simulink model "CM012A_FordT3McuCfg"  (R2013b)
settings: Solver=FixedStepDiscrete  SolverMode=SingleTasking  StartTime=0.0  StopTime=2  FixedStep=0.00005  RelTol=1e-3
values from neighbouring files (symbols this model uses):
  BATTVLTGSCAGFAC_ULS_F32 = DataDict.Constant    [CM012A_FordT3McuCfg_DataDict.m]
  BATTVLTGSWD1SCAGFAC_ULS_F32 = DataDict.Constant    [CM012A_FordT3McuCfg_DataDict.m]
  CHRGPMPDIAGSCAGFAC_ULS_F32 = DataDict.Constant    [CM012A_FordT3McuCfg_DataDict.m]
  MOTAG2MEAS_ECU1OFFS_MOTREV_F32 = DataDict.Constant    [CM012A_FordT3McuCfg_DataDict.m]
  MOTAG2MEAS_ECU2OFFS_MOTREV_F32 = DataDict.Constant    [CM012A_FordT3McuCfg_DataDict.m]
  PWRDISCNCTSWTDIAGSCAGFAC_ULS_F32 = DataDict.Constant    [CM012A_FordT3McuCfg_DataDict.m]
undefined symbols (not defined in the file or in its folder): HwAgSnsrTyp1, sigbuilder_block
libraries: CM012A_FordT3McuCfg_ModelLibrary x114, simulink x37, NxtrLim x34
(part 2 of 4)

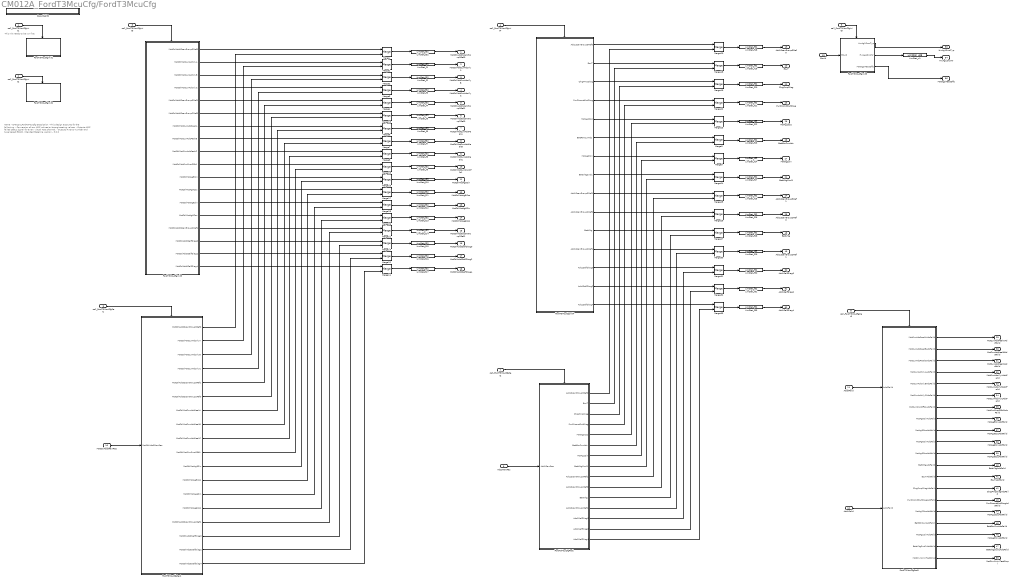
== system CM012A_FordT3McuCfg/FordT3McuCfg ==
  note: Name - 		CM012A_FordT3McuCfg
      | Description -  This design accounts for the following,
      | 			- Conversion of raw ADC values to its engineering values.
      | 			- Outputs ADC failed status signal for every virtual ADC channel.
      | 			- Outputs HwSnsr number and type based ECUID.
      | Intended Baseline version - 3.0.0
  note: This Init needs to be run first
  call_FordT3McuCfgInit1 : Inport
  call_FordT3McuCfgInit2 : Inport  Port=2
  call_FordT3McuCfgInit3 : Inport  Port=3
  call_FordT3McuCfgInit4 : Inport  Port=4
  call_FordT3McuCfgInit5 : Inport  Port=5
  call_FordT3McuCfgPer1 : Inport  Port=6
  call_FordT3McuCfgPer2 : Inport  Port=7
  call_FordT3McuCfgPer3 : Inport  Port=8
  Adc1RawRes : Inport  RequirementInfo="{'linktype_rmi_doors' '00016ba8 (/ESG Group/FDD Module Requirements/EA4 Specific/CM012A_FordT3McuCfg)' '#CM012A_80' 'true' 'REQ:  CM012A_80' '' } %GIDa_41160691_1e7a_406c_957b_4d6a456ee094"  Port=9
  MotCtrlAdc0RawRes : Inport  RequirementInfo="{'linktype_rmi_doors' '00016ba8 (/ESG Group/FDD Module Requirements/EA4 Specific/CM012A_FordT3McuCfg)' '#CM012A_30' 'true' 'REQ:  CM012A_30' '' } %GIDa_99229d35_45d9_4e08_a805_76e263dac1ca"  Port=10
  Adc0Faild : Inport  RequirementInfo="{'linktype_rmi_doors' '00016ba8 (/ESG Group/FDD Module Requirements/EA4 Specific/CM012A_FordT3McuCfg)' '#CM012A_108' 'true' 'REQ:  CM012A_108' '' } %GIDa_0bce0144_3b89_427c_817c_6b44de9e7a17"  Port=11
  Adc1Faild : Inport  RequirementInfo="{'linktype_rmi_doors' '00016ba8 (/ESG Group/FDD Module Requirements/EA4 Specific/CM012A_FordT3McuCfg)' '#CM012A_109' 'true' 'REQ:  CM012A_109' '' } %GIDa_dca9ee74_b82a_443a_9b96_53a5f3cd54c7"  Port=12
  EcuId : Inport  RequirementInfo="{'linktype_rmi_doors' '00016ba8 (/ESG Group/FDD Module Requirements/EA4 Specific/CM012A_FordT3McuCfg)' '#CM012A_110' 'true' 'REQ:  CM012A_110' '' } %GIDa_2ea2a6bb_1285_46d2_bb52_886e41c9a838"  Port=13
  CopyRight2 : Subsystem  Description=|  mask(Copyright Information){none=on}
      | Copyright info block.                                               
      |                                                                     
      | Place copyright information at the top of every subsystem in design.
      mask prompts: none "No parameters"
      mask help: Place copyright information at the top of every subsystem in design.
      mask Display:
      | NxtrConf = 'Nexteer Confidential';
      | 
      | sys = bdroot; %handle for the current model ("system")
      | first = get_param(sys,'Created');
      | first = first(end-3:end);  %year is last four digits
      | 
      | last = get_param(sys,'LastModifiedDate');
      | if isempty(last)
      |     last = datestr(now,'yyyy');
      | else
      |     last = last(end-3:end);
      | end
      | 
      | if strcmp(first,last)
      |     fprintf('%s -- Copyright %s Nexteer',NxtrConf,first)
      | else
      |     fprintf('%s -- %s%s- %s Nexteer',NxtrConf,char(169),first,last)
      | end
  FordT3McuCfgInit1 : Subsystem
  FordT3McuCfgInit2 : Subsystem
  FordT3McuCfgInit3 : Subsystem
  FordT3McuCfgInit4 : Subsystem
  FordT3McuCfgInit5 : Subsystem  RequirementInfo="{'linktype_rmi_doors' '00016ba8 (/ESG Group/FDD Module Requirements/EA4 Specific/CM012A_FordT3McuCfg)' '#CM012A_188' 'true' 'REQ:  CM012A_188' '' } %GIDa_a4501015_2e8d_4379_8b64_871cd7f02fc6"
  FordT3McuCfgPer1 : Subsystem  RequirementInfo="{'linktype_rmi_doors' '00016ba8 (/ESG Group/FDD Module Requirements/EA4 Specific/CM012A_FordT3McuCfg)' '#CM012A_113' 'true' 'REQ:  CM012A_113' '' } %GIDa_f4084d5f_812f_4f7b_9c4a_edd3fedcd563"
      settings: AttributesFormatString=Priority: %<Priority>
  FordT3McuCfgPer2 : Subsystem  RequirementInfo="{'linktype_rmi_doors' '00016ba8 (/ESG Group/FDD Module Requirements/EA4 Specific/CM012A_FordT3McuCfg)' '#CM012A_114' 'true' 'REQ:  CM012A_114' '' } %GIDa_f8eec309_27b4_4df0_b18c_c2951f94362c"
      settings: AttributesFormatString=Priority: %<Priority>
  FordT3McuCfgPer3 : Subsystem  RequirementInfo="{'linktype_rmi_doors' '00016ba8 (/ESG Group/FDD Module Requirements/EA4 Specific/CM012A_FordT3McuCfg)' '#CM012A_134' 'true' 'REQ:  CM012A_134' '' } %GIDa_f61b09d0_e9f4_4379_bee3_c878705b543d"
      settings: AttributesFormatString=Priority: %<Priority>
  LimStat_f{1..19,22..26,29..33} (29 alike) : NxtrLim/LimStat_f32  LoLim=0  HiLim=ADCOUTPMAX_VOLT_F32
      settings: AttributesFormatString=|
      | Low Limit: %<LoLim>
      | High Limit:%<HiLim>
  LimStat_f{20..21,27..28} (4 alike) : NxtrLim/LimStat_f32  LoLim=0  HiLim=BATTADCOUTPMAX_VOLT_F32
      settings: AttributesFormatString=|
      | Low Limit: %<LoLim>
      | High Limit:%<HiLim>
  LimStat_u1 : NxtrLim/LimStat_u08  LoLim=0  HiLim=HWAG1SNSRNRMAX_CNT_F32
      settings: AttributesFormatString=|
      | Low Limit: %<LoLim>
      | High Limit:%<HiLim>
  Merge{,1..9,11..33} (33 alike) : Merge
  MotCtrlAdc0ScanGroup3Ref0 : Outport
  MotCtrlMotCurrAdcVlyA : Outport  RequirementInfo="{'linktype_rmi_doors' '00016ba8 (/ESG Group/FDD Module Requirements/EA4 Specific/CM012A_FordT3McuCfg)' '#CM012A_31' 'true' 'REQ:  CM012A_31' '' } %GIDa_0bdba440_75b6_48b6_84a8_aedbc0ed0aee"  Port=2
  MotCtrlMotCurrAdcVlyB : Outport  RequirementInfo="{'linktype_rmi_doors' '00016ba8 (/ESG Group/FDD Module Requirements/EA4 Specific/CM012A_FordT3McuCfg)' '#CM012A_97' 'true' 'REQ:  CM012A_97' '' } %GIDa_ce9d7107_8d39_410b_aef3_5c211a563983"  Port=3
  MotCtrlMotCurrAdcVlyC : Outport  RequirementInfo="{'linktype_rmi_doors' '00016ba8 (/ESG Group/FDD Module Requirements/EA4 Specific/CM012A_FordT3McuCfg)' '#CM012A_96' 'true' 'REQ:  CM012A_96' '' } %GIDa_d8883527_c83e_4baa_9ea4_71e3d2339800"  Port=4
  MotCtrlAdc0ScanGroup3Ref1 : Outport  Port=5
  MotCtrlAdc0ScanGroup2Ref0 : Outport  Port=6
  MotCtrlMotCurrAdcPeakA : Outport  RequirementInfo="{'linktype_rmi_doors' '00016ba8 (/ESG Group/FDD Module Requirements/EA4 Specific/CM012A_FordT3McuCfg)' '#CM012A_135' 'true' 'REQ:  CM012A_135' '' } %GIDa_3269826c_f262_49f9_8a60_4071384b86b7"  Port=7
  MotCtrlMotCurrAdcPeakB : Outport  RequirementInfo="{'linktype_rmi_doors' '00016ba8 (/ESG Group/FDD Module Requirements/EA4 Specific/CM012A_FordT3McuCfg)' '#CM012A_136' 'true' 'REQ:  CM012A_136' '' } %GIDa_7e88d78e_c6ec_4e32_98f2_6110e77972ae"  Port=8
  MotCtrlMotCurrAdcPeakC : Outport  RequirementInfo="{'linktype_rmi_doors' '00016ba8 (/ESG Group/FDD Module Requirements/EA4 Specific/CM012A_FordT3McuCfg)' '#CM012A_137' 'true' 'REQ:  CM012A_137' '' } %GIDa_58277148_ccdb_4560_8c9d_d26260a4df88"  Port=9
  MotCtrlMotCurrSnsrOffs1 : Outport  RequirementInfo="{'linktype_rmi_doors' '00016ba8 (/ESG Group/FDD Module Requirements/EA4 Specific/CM012A_FordT3McuCfg)' '#CM012A_138' 'true' 'REQ:  CM012A_138' '' } %GIDa_8dfc8efb_0597_44a1_ac28_cdaba55153cb"  Port=10
  MotCtrlMotAg5Sin : Outport  RequirementInfo="{'linktype_rmi_doors' '00016ba8 (/ESG Group/FDD Module Requirements/EA4 Specific/CM012A_FordT3McuCfg)' '#CM012A_139' 'true' 'REQ:  CM012A_139' '' } %GIDa_8814a36d_2960_4cab_9305_7cef514a95a4"  Port=11
  MotCtrlMotAg5Cos : Outport  RequirementInfo="{'linktype_rmi_doors' '00016ba8 (/ESG Group/FDD Module Requirements/EA4 Specific/CM012A_FordT3McuCfg)' '#CM012A_140' 'true' 'REQ:  CM012A_140' '' } %GIDa_cf319651_e51f_428f_a8b0_82c784d893cb"  Port=12
  MotCtrlMotAg6Sin : Outport  RequirementInfo="{'linktype_rmi_doors' '00016ba8 (/ESG Group/FDD Module Requirements/EA4 Specific/CM012A_FordT3McuCfg)' '#CM012A_141' 'true' 'REQ:  CM012A_141' '' } %GIDa_f3249900_9d1e_416f_98e2_ff7658e30e7b"  Port=13
  MotCtrlMotAg6Cos : Outport  RequirementInfo="{'linktype_rmi_doors' '00016ba8 (/ESG Group/FDD Module Requirements/EA4 Specific/CM012A_FordT3McuCfg)' '#CM012A_142' 'true' 'REQ:  CM012A_142' '' } %GIDa_bed7064b_f1cf_47a3_89f1_2e6806942a9b"  Port=14
  MotCtrlAdc0ScanGroup2Ref1 : Outport  Port=15
  MotCtrlAdc0SelfDiag0 : Outport  Port=16
  MotCtrlAdc0SelfDiag2 : Outport  Port=17
  MotCtrlAdc0SelfDiag4 : Outport  Port=18
  Adc1ScanGroup3Ref0 : Outport  Port=19
  EcuT : Outport  RequirementInfo="{'linktype_rmi_doors' '00016ba8 (/ESG Group/FDD Module Requirements/EA4 Specific/CM012A_FordT3McuCfg)' '#CM012A_143' 'true' 'REQ:  CM012A_143' '' } %GIDa_4e0089fd_73ae_4216_9e55_f5e900769cc9"  Port=20
  BattVltgSwd1 : Outport  RequirementInfo="{'linktype_rmi_doors' '00016ba8 (/ESG Group/FDD Module Requirements/EA4 Specific/CM012A_FordT3McuCfg)' '#CM012A_148' 'true' 'REQ:  CM012A_148' '' } %GIDa_a4fbd9dd_cc02_44b6_8c60_edd2cbad70c3"  Port=21
  ChrgPmpDiag : Outport  RequirementInfo="{'linktype_rmi_doors' '00016ba8 (/ESG Group/FDD Module Requirements/EA4 Specific/CM012A_FordT3McuCfg)' '#CM012A_144' 'true' 'REQ:  CM012A_144' '' } %GIDa_9af4aaf1_e6d4_4150_aa90_b727a20d0e65"  Port=22
  PwrDiscnctSwtDiag : Outport  RequirementInfo="{'linktype_rmi_doors' '00016ba8 (/ESG Group/FDD Module Requirements/EA4 Specific/CM012A_FordT3McuCfg)' '#CM012A_186' 'true' 'REQ:  CM012A_186' '' } %GIDa_25930d50_606d_4173_986f_d131b07fb4a3"  Port=23
  Adc1ScanGroup3Ref1 : Outport  Port=24
  Adc1ScanGroup2Ref0 : Outport  Port=25
  MotAg2Cos : Outport  RequirementInfo="{'linktype_rmi_doors' '00016ba8 (/ESG Group/FDD Module Requirements/EA4 Specific/CM012A_FordT3McuCfg)' '#CM012A_145' 'true' 'REQ:  CM012A_145' '' } %GIDa_fb1722b1_4d2c_4680_9aaf_1a870d66429d"  Port=26
  MotAg2Sin : Outport  RequirementInfo="{'linktype_rmi_doors' '00016ba8 (/ESG Group/FDD Module Requirements/EA4 Specific/CM012A_FordT3McuCfg)' '#CM012A_147' 'true' 'REQ:  CM012A_147' '' } %GIDa_119a92d6_b549_4670_801c_893abfbf86fb"  Port=27
  BattRtnCurrAdc : Outport  RequirementInfo="{'linktype_rmi_doors' '00016ba8 (/ESG Group/FDD Module Requirements/EA4 Specific/CM012A_FordT3McuCfg)' '#CM012A_146' 'true' 'REQ:  CM012A_146' '' } %GIDa_bf47c31e_57b3_45f9_b1b7_bf963f3d70ff"  Port=28
  MotCurrAdcPeakAAdcFaild : Outport  RequirementInfo="{'linktype_rmi_doors' '00016ba8 (/ESG Group/FDD Module Requirements/EA4 Specific/CM012A_FordT3McuCfg)' '#CM012A_149' 'true' 'REQ:  CM012A_149' '' } %GIDa_3a53e3dd_f880_4695_94e7_22bc9fe6702f"  Port=29
  MotCurrAdcPeakBAdcFaild : Outport  RequirementInfo="{'linktype_rmi_doors' '00016ba8 (/ESG Group/FDD Module Requirements/EA4 Specific/CM012A_FordT3McuCfg)' '#CM012A_150' 'true' 'REQ:  CM012A_150' '' } %GIDa_feafdf78_53ff_40fe_9421_17b92296df86"  Port=30
  MotCurrAdcPeakCAdcFaild : Outport  RequirementInfo="{'linktype_rmi_doors' '00016ba8 (/ESG Group/FDD Module Requirements/EA4 Specific/CM012A_FordT3McuCfg)' '#CM012A_151' 'true' 'REQ:  CM012A_151' '' } %GIDa_56e34d84_3367_4a32_8cb7_70a413310ee9"  Port=31
  MotCurrAdcVlyAAdcFaild : Outport  RequirementInfo="{'linktype_rmi_doors' '00016ba8 (/ESG Group/FDD Module Requirements/EA4 Specific/CM012A_FordT3McuCfg)' '#CM012A_152' 'true' 'REQ:  CM012A_152' '' } %GIDa_235f97ec_d780_48fb_a6ee_f7442017c90d"  Port=32
  MotCurrAdcVlyBAdcFaild : Outport  RequirementInfo="{'linktype_rmi_doors' '00016ba8 (/ESG Group/FDD Module Requirements/EA4 Specific/CM012A_FordT3McuCfg)' '#CM012A_153' 'true' 'REQ:  CM012A_153' '' } %GIDa_353b0153_747a_4ed6_88df_12a4ad6b71ec"  Port=33
  MotCurrAdcVlyCAdcFaild : Outport  RequirementInfo="{'linktype_rmi_doors' '00016ba8 (/ESG Group/FDD Module Requirements/EA4 Specific/CM012A_FordT3McuCfg)' '#CM012A_154' 'true' 'REQ:  CM012A_154' '' } %GIDa_a57b872d_9b77_463d_8457_590115cc1f58"  Port=34
  MotCurrSnsrOffs1AdcFaild : Outport  RequirementInfo="{'linktype_rmi_doors' '00016ba8 (/ESG Group/FDD Module Requirements/EA4 Specific/CM012A_FordT3McuCfg)' '#CM012A_155' 'true' 'REQ:  CM012A_155' '' } %GIDa_dab1b948_9138_4007_9c31_06f0147cb8f7"  Port=35
  MotAg5SinAdcFaild : Outport  RequirementInfo="{'linktype_rmi_doors' '00016ba8 (/ESG Group/FDD Module Requirements/EA4 Specific/CM012A_FordT3McuCfg)' '#CM012A_156' 'true' 'REQ:  CM012A_156' '' } %GIDa_0b267258_9b4b_4074_b8ac_2e562917866b"  Port=36
  MotAg5CosAdcFaild : Outport  RequirementInfo="{'linktype_rmi_doors' '00016ba8 (/ESG Group/FDD Module Requirements/EA4 Specific/CM012A_FordT3McuCfg)' '#CM012A_157' 'true' 'REQ:  CM012A_157' '' } %GIDa_2a7f7a18_8db2_45e1_a969_e1b831e06969"  Port=37
  MotAg6SinAdcFaild : Outport  RequirementInfo="{'linktype_rmi_doors' '00016ba8 (/ESG Group/FDD Module Requirements/EA4 Specific/CM012A_FordT3McuCfg)' '#CM012A_158' 'true' 'REQ:  CM012A_158' '' } %GIDa_5066297d_e1ca_466f_b5fd_4f065ba4d243"  Port=38
  MotAg6CosAdcFaild : Outport  RequirementInfo="{'linktype_rmi_doors' '00016ba8 (/ESG Group/FDD Module Requirements/EA4 Specific/CM012A_FordT3McuCfg)' '#CM012A_159' 'true' 'REQ:  CM012A_159' '' } %GIDa_42b69db8_ef47_41c4_a15d_6b9505077de8"  Port=39
  BattVltgAdcFaild : Outport  RequirementInfo="{'linktype_rmi_doors' '00016ba8 (/ESG Group/FDD Module Requirements/EA4 Specific/CM012A_FordT3McuCfg)' '#CM012A_160' 'true' 'REQ:  CM012A_160' '' } %GIDa_f2237051_f0a5_4ae7_a3b8_c07d1c352a88"  Port=40
  EcuTAdcFaild : Outport  RequirementInfo="{'linktype_rmi_doors' '00016ba8 (/ESG Group/FDD Module Requirements/EA4 Specific/CM012A_FordT3McuCfg)' '#CM012A_161' 'true' 'REQ:  CM012A_161' '' } %GIDa_f8c196a4_34a8_4792_9bba_d1d568e93057"  Port=41
  ChrgPmpDiagAdcFaild : Outport  RequirementInfo="{'linktype_rmi_doors' '00016ba8 (/ESG Group/FDD Module Requirements/EA4 Specific/CM012A_FordT3McuCfg)' '#CM012A_162' 'true' 'REQ:  CM012A_162' '' } %GIDa_77beee14_d374_44df_95fc_54a895c9cfa9"  Port=42
  PwrDiscnctSwtDiagAdcFaild : Outport  RequirementInfo="{'linktype_rmi_doors' '00016ba8 (/ESG Group/FDD Module Requirements/EA4 Specific/CM012A_FordT3McuCfg)' '#CM012A_163' 'true' 'REQ:  CM012A_163' '' } %GIDa_31860440_5fb5_4509_8c25_9f6b0fdcba7a"  Port=43
  MotAg2CosAdcFaild : Outport  RequirementInfo="{'linktype_rmi_doors' '00016ba8 (/ESG Group/FDD Module Requirements/EA4 Specific/CM012A_FordT3McuCfg)' '#CM012A_164' 'true' 'REQ:  CM012A_164' '' } %GIDa_a152779b_3d52_4dd5_9e9f_688e8ab12150"  Port=44
  BattRtnCurrAdcFaild : Outport  RequirementInfo="{'linktype_rmi_doors' '00016ba8 (/ESG Group/FDD Module Requirements/EA4 Specific/CM012A_FordT3McuCfg)' '#CM012A_165' 'true' 'REQ:  CM012A_165' '' } %GIDa_209c41ad_d5d9_4f94_9c3e_4b63790d466d"  Port=45
  MotAg2SinAdcFaild : Outport  RequirementInfo="{'linktype_rmi_doors' '00016ba8 (/ESG Group/FDD Module Requirements/EA4 Specific/CM012A_FordT3McuCfg)' '#CM012A_166' 'true' 'REQ:  CM012A_166' '' } %GIDa_2107ec05_8c9a_4950_b739_abe494ef6948"  Port=46
  BattVltgSwd1AdcFaild : Outport  RequirementInfo="{'linktype_rmi_doors' '00016ba8 (/ESG Group/FDD Module Requirements/EA4 Specific/CM012A_FordT3McuCfg)' '#CM012A_167' 'true' 'REQ:  CM012A_167' '' } %GIDa_c3b1591d_1c63_48f3_97b0_16e822f187b4"  Port=47
  BattVltg : Outport  RequirementInfo="{'linktype_rmi_doors' '00016ba8 (/ESG Group/FDD Module Requirements/EA4 Specific/CM012A_FordT3McuCfg)' '#CM012A_187' 'true' 'REQ:  CM012A_187' '' } %GIDa_e1d6f2ac_b011_4b4e_acb7_aa6bb65164ac"  Port=48
  Adc1ScanGroup2Ref1 : Outport  Port=49
  Adc1SelfDiag0 : Outport  Port=50
  Adc1SelfDiag2 : Outport  Port=51
  Adc1SelfDiag4 : Outport  Port=52
  HwAg1SnsrTyp : Outport  RequirementInfo="{'linktype_rmi_doors' '00016ba8 (/ESG Group/FDD Module Requirements/EA4 Specific/CM012A_FordT3McuCfg)' '#CM012A_168' 'true' 'REQ:  CM012A_168' '' } %GIDa_345868f1_11a8_4efe_8557_e97fce4612b7"  Port=53
  HwAg1SnsrNr : Outport  RequirementInfo="{'linktype_rmi_doors' '00016ba8 (/ESG Group/FDD Module Requirements/EA4 Specific/CM012A_FordT3McuCfg)' '#CM012A_169' 'true' 'REQ:  CM012A_169' '' } %GIDa_0d5e4ab3_9e68_4afd_8e94_0b3421e961a0"  Port=54
  MotDrvr1IninTestCmpl : Outport  Port=55
  MotAg2MeasOffs : Outport  RequirementInfo="{'linktype_rmi_doors' '00016ba8 (/ESG Group/FDD Module Requirements/EA4 Specific/CM012A_FordT3McuCfg)' '#CM012A_192' 'true' 'REQ:  CM012A_192' '' } %GIDa_2a555be6_74a0_4831_8830_82a88131d4c1"  Port=56
  wires:
  FordT3McuCfgInit3/1(MotCtrlAdc0ScanGroup3Ref0) -> Merge/1
  FordT3McuCfgInit3/2(MotCtrlMotCurrAdcVlyA) -> Merge1/1
  FordT3McuCfgInit3/3(MotCtrlMotCurrAdcVlyB) -> Merge2/1
  FordT3McuCfgInit3/4(MotCtrlMotCurrAdcVlyC) -> Merge3/1
  FordT3McuCfgInit3/5(MotCtrlAdc0ScanGroup3Ref1) -> Merge4/1
  FordT3McuCfgInit3/6(MotCtrlAdc0ScanGroup2Ref0) -> Merge13/1
  FordT3McuCfgInit3/7(MotCtrlMotCurrAdcPeakA) -> Merge6/1
  FordT3McuCfgInit3/8(MotCtrlMotCurrAdcPeakB) -> Merge7/1
  FordT3McuCfgInit3/9(MotCtrlMotCurrAdcPeakC) -> Merge8/1
  FordT3McuCfgInit3/10(MotCtrlMotCurrSnsrOffs1) -> Merge15/1
  FordT3McuCfgInit3/11(MotCtrlMotAg5Sin) -> Merge16/1
  FordT3McuCfgInit3/12(MotCtrlMotAg5Cos) -> Merge17/1
  FordT3McuCfgInit3/13(MotCtrlMotAg6Sin) -> Merge28/1
  FordT3McuCfgInit3/14(MotCtrlMotAg6Cos) -> Merge26/1
  FordT3McuCfgInit3/15(MotCtrlAdc0ScanGroup2Ref1) -> Merge21/1
  FordT3McuCfgInit3/16(MotCtrlAdc0SelfDiag0) -> Merge14/1
  FordT3McuCfgInit3/17(MotCtrlAdc0SelfDiag2) -> Merge12/1
  FordT3McuCfgInit3/18(MotCtrlAdc0SelfDiag4) -> Merge11/1
  FordT3McuCfgPer1/18(MotCtrlAdc0SelfDiag4) -> Merge11/2
  FordT3McuCfgPer1/17(MotCtrlAdc0SelfDiag2) -> Merge12/2
  FordT3McuCfgPer1/16(MotCtrlAdc0SelfDiag0) -> Merge14/2
  FordT3McuCfgPer1/15(MotCtrlAdc0ScanGroup2Ref1) -> Merge21/2
  FordT3McuCfgPer1/14(MotCtrlMotAg6Cos) -> Merge26/2
  FordT3McuCfgPer1/13(MotCtrlMotAg6Sin) -> Merge28/2
  FordT3McuCfgPer1/12(MotCtrlMotAg5Cos) -> Merge17/2
  FordT3McuCfgPer1/11(MotCtrlMotAg5Sin) -> Merge16/2
  FordT3McuCfgPer1/10(MotCtrlMotCurrSnsrOffs1) -> Merge15/2
  FordT3McuCfgPer1/9(MotCtrlMotCurrAdcPeakC) -> Merge8/2
  FordT3McuCfgPer1/8(MotCtrlMotCurrAdcPeakB) -> Merge7/2
  FordT3McuCfgPer1/7(MotCtrlMotCurrAdcPeakA) -> Merge6/2
  Merge/1 -> LimStat_f32/1
  Merge1/1 -> LimStat_f1/1
  Merge2/1 -> LimStat_f2/1
  Merge3/1 -> LimStat_f3/1
  Merge4/1 -> LimStat_f4/1
  Merge13/1 -> LimStat_f5/1
  Merge6/1 -> LimStat_f6/1
  Merge7/1 -> LimStat_f7/1
  Merge8/1 -> LimStat_f8/1
  Merge15/1 -> LimStat_f9/1
  Merge16/1 -> LimStat_f10/1
  Merge26/1 -> LimStat_f13/1
  Merge28/1 -> LimStat_f12/1
  Merge17/1 -> LimStat_f11/1
  Merge21/1 -> LimStat_f14/1
  Merge14/1 -> LimStat_f15/1
  Merge11/1 -> LimStat_f17/1
  Merge12/1 -> LimStat_f16/1
  FordT3McuCfgPer1/6(MotCtrlAdc0ScanGroup2Ref0) -> Merge13/2
  FordT3McuCfgPer1/5(MotCtrlAdc0ScanGroup3Ref1) -> Merge4/2
  FordT3McuCfgPer1/4(MotCtrlMotCurrAdcVlyC) -> Merge3/2
  FordT3McuCfgPer1/3(MotCtrlMotCurrAdcVlyB) -> Merge2/2
  FordT3McuCfgPer1/2(MotCtrlMotCurrAdcVlyA) -> Merge1/2
  FordT3McuCfgPer1/1(MotCtrlAdc0ScanGroup3Ref0) -> Merge/2
  Merge20/1 -> LimStat_f18/1
  Merge18/1 -> LimStat_f19/1
  Merge24/1 -> LimStat_f27/1
  Merge19/1 -> LimStat_f20/1
  Merge22/1 -> LimStat_f21/1
  Merge25/1 -> LimStat_f25/1
  Merge29/1 -> LimStat_f26/1
  Merge23/1 -> LimStat_f22/1
  Merge9/1 -> LimStat_f24/1
  Merge5/1 -> LimStat_f23/1
  FordT3McuCfgPer3/11(MotAg6CosAdcFaild) -> MotAg6CosAdcFaild/1
  FordT3McuCfgPer3/10(MotAg6SinAdcFaild) -> MotAg6SinAdcFaild/1
  FordT3McuCfgPer3/9(MotAg5CosAdcFaild) -> MotAg5CosAdcFaild/1
  FordT3McuCfgPer3/8(MotAg5SinAdcFaild) -> MotAg5SinAdcFaild/1
  FordT3McuCfgPer3/7(MotCurrSnsrOffs1AdcFaild) -> MotCurrSnsrOffs1AdcFaild/1
  FordT3McuCfgPer3/6(MotCurrAdcVlyCAdcFaild) -> MotCurrAdcVlyCAdcFaild/1
  FordT3McuCfgPer3/5(MotCurrAdcVlyBAdcFaild) -> MotCurrAdcVlyBAdcFaild/1
  FordT3McuCfgPer3/4(MotCurrAdcVlyAAdcFaild) -> MotCurrAdcVlyAAdcFaild/1
  FordT3McuCfgPer3/3(MotCurrAdcPeakCAdcFaild) -> MotCurrAdcPeakCAdcFaild/1
  FordT3McuCfgPer3/2(MotCurrAdcPeakBAdcFaild) -> MotCurrAdcPeakBAdcFaild/1
  FordT3McuCfgPer3/1(MotCurrAdcPeakAAdcFaild) -> MotCurrAdcPeakAAdcFaild/1
  FordT3McuCfgPer3/12(BattVltgAdcFaild) -> BattVltgAdcFaild/1
  FordT3McuCfgPer3/13(EcuTAdcFaild) -> EcuTAdcFaild/1
  FordT3McuCfgPer3/14(ChrgPmpDiagAdcFaild) -> ChrgPmpDiagAdcFaild/1
  FordT3McuCfgPer3/15(PwrDiscnctSwtDiagAdcFaild) -> PwrDiscnctSwtDiagAdcFaild/1
  FordT3McuCfgPer3/16(MotAg2CosAdcFaild) -> MotAg2CosAdcFaild/1
  FordT3McuCfgPer3/17(BattRtnCurrAdcFaild) -> BattRtnCurrAdcFaild/1
  FordT3McuCfgPer3/18(MotAg2SinAdcFaild) -> MotAg2SinAdcFaild/1
  FordT3McuCfgPer3/19(BattVltgSwd1AdcFaild) -> BattVltgSwd1AdcFaild/1
  Merge27/1 -> LimStat_f28/1
  Merge30/1 -> LimStat_f29/1
  Merge33/1 -> LimStat_f33/1
  Merge32/1 -> LimStat_f31/1
  Merge31/1 -> LimStat_f30/1
  FordT3McuCfgInit4/1(Adc1ScanGroup3Ref0) -> Merge20/1
  FordT3McuCfgInit4/2(EcuT) -> Merge18/1
  FordT3McuCfgInit4/3(ChrgPmpDiag) -> Merge19/1
  FordT3McuCfgInit4/4(PwrDiscnctSwtDiag) -> Merge22/1
  FordT3McuCfgInit4/5(MotAg2Cos) -> Merge23/1
  FordT3McuCfgInit4/6(BattRtnCurrAdc) -> Merge5/1
  FordT3McuCfgInit4/7(MotAg2Sin) -> Merge9/1
  FordT3McuCfgInit4/8(BattVltgSwd1) -> Merge24/1
  FordT3McuCfgInit4/9(Adc1ScanGroup3Ref1) -> Merge25/1
  FordT3McuCfgInit4/10(Adc1ScanGroup2Ref0) -> Merge29/1
  FordT3McuCfgInit4/11(BattVltg) -> Merge27/1
  FordT3McuCfgInit4/12(Adc1ScanGroup2Ref1) -> Merge30/1
  FordT3McuCfgInit4/13(Adc1SelfDiag0) -> Merge31/1
  FordT3McuCfgInit4/14(Adc1SelfDiag2) -> Merge32/1
  FordT3McuCfgInit4/15(Adc1SelfDiag4) -> Merge33/1
  FordT3McuCfgPer2/15(Adc1SelfDiag4) -> Merge33/2
  FordT3McuCfgPer2/14(Adc1SelfDiag2) -> Merge32/2
  FordT3McuCfgPer2/13(Adc1SelfDiag0) -> Merge31/2
  FordT3McuCfgPer2/12(Adc1ScanGroup2Ref1) -> Merge30/2
  FordT3McuCfgPer2/11(BattVltg) -> Merge27/2
  FordT3McuCfgPer2/10(Adc1ScanGroup2Ref0) -> Merge29/2
  FordT3McuCfgPer2/9(Adc1ScanGroup3Ref1) -> Merge25/2
  FordT3McuCfgPer2/8(BattVltgSwd1) -> Merge24/2
  FordT3McuCfgPer2/7(MotAg2Sin) -> Merge9/2
  FordT3McuCfgPer2/6(BattRtnCurrAdc) -> Merge5/2
  FordT3McuCfgPer2/5(MotAg2Cos) -> Merge23/2
  FordT3McuCfgPer2/4(PwrDiscnctSwtDiag) -> Merge22/2
  FordT3McuCfgPer2/3(ChrgPmpDiag) -> Merge19/2
  FordT3McuCfgPer2/2(EcuT) -> Merge18/2
  FordT3McuCfgPer2/1(Adc1ScanGroup3Ref0) -> Merge20/2
  FordT3McuCfgInit5/2(HwAg1SnsrNr) -> LimStat_u1/1
  LimStat_f32/1 -> MotCtrlAdc0ScanGroup3Ref0/1
  LimStat_f1/1 -> MotCtrlMotCurrAdcVlyA/1
  LimStat_f2/1 -> MotCtrlMotCurrAdcVlyB/1
  LimStat_f3/1 -> MotCtrlMotCurrAdcVlyC/1
  LimStat_f4/1 -> MotCtrlAdc0ScanGroup3Ref1/1
  LimStat_f5/1 -> MotCtrlAdc0ScanGroup2Ref0/1
  LimStat_f6/1 -> MotCtrlMotCurrAdcPeakA/1
  LimStat_f7/1 -> MotCtrlMotCurrAdcPeakB/1
  LimStat_f8/1 -> MotCtrlMotCurrAdcPeakC/1
  LimStat_f9/1 -> MotCtrlMotCurrSnsrOffs1/1
  LimStat_f10/1 -> MotCtrlMotAg5Sin/1
  LimStat_f11/1 -> MotCtrlMotAg5Cos/1
  LimStat_f12/1 -> MotCtrlMotAg6Sin/1
  LimStat_f13/1 -> MotCtrlMotAg6Cos/1
  LimStat_f14/1 -> MotCtrlAdc0ScanGroup2Ref1/1
  LimStat_f15/1 -> MotCtrlAdc0SelfDiag0/1
  LimStat_f16/1 -> MotCtrlAdc0SelfDiag2/1
  LimStat_f17/1 -> MotCtrlAdc0SelfDiag4/1
  LimStat_f18/1 -> Adc1ScanGroup3Ref0/1
  LimStat_f19/1 -> EcuT/1
  LimStat_f20/1 -> ChrgPmpDiag/1
  LimStat_f21/1 -> PwrDiscnctSwtDiag/1
  LimStat_f22/1 -> MotAg2Cos/1
  LimStat_f23/1 -> BattRtnCurrAdc/1
  LimStat_f24/1 -> MotAg2Sin/1
  LimStat_f25/1 -> Adc1ScanGroup3Ref1/1
  LimStat_f26/1 -> Adc1ScanGroup2Ref0/1
  LimStat_f27/1 -> BattVltgSwd1/1
  LimStat_f28/1 -> BattVltg/1
  LimStat_f29/1 -> Adc1ScanGroup2Ref1/1
  LimStat_f30/1 -> Adc1SelfDiag0/1
  LimStat_f31/1 -> Adc1SelfDiag2/1
  LimStat_f33/1 -> Adc1SelfDiag4/1
  FordT3McuCfgInit5/1(HwAg1SnsrTyp) -> HwAg1SnsrTyp/1
  LimStat_u1/1 -> HwAg1SnsrNr/1
  call_FordT3McuCfgInit1/1 -> FordT3McuCfgInit1/Trigger
  FordT3McuCfgPer3/20(MotDrvr1IninTestCmpl) -> MotDrvr1IninTestCmpl/1
  call_FordT3McuCfgInit2/1 -> FordT3McuCfgInit2/Trigger
  call_FordT3McuCfgInit3/1 -> FordT3McuCfgInit3/Trigger
  call_FordT3McuCfgInit4/1 -> FordT3McuCfgInit4/Trigger
  call_FordT3McuCfgInit5/1 -> FordT3McuCfgInit5/Trigger
  call_FordT3McuCfgPer1/1 -> FordT3McuCfgPer1/Trigger
  call_FordT3McuCfgPer2/1 -> FordT3McuCfgPer2/Trigger
  call_FordT3McuCfgPer3/1 -> FordT3McuCfgPer3/Trigger
  Adc1RawRes/1 -> FordT3McuCfgPer2/1(Adc1RawRes)
  MotCtrlAdc0RawRes/1 -> FordT3McuCfgPer1/1(MotCtrlAdc0RawRes)
  Adc0Faild/1 -> FordT3McuCfgPer3/1(Adc0Faild)
  Adc1Faild/1 -> FordT3McuCfgPer3/2(Adc1Faild)
  EcuId/1 -> FordT3McuCfgInit5/1(EcuId)
  FordT3McuCfgInit5/3(MotAg2MeasOffs) -> MotAg2MeasOffs/1

== system CM012A_FordT3McuCfg/Signal Builder ==
  Demux : Demux  Tag=STV Demux  Outputs=1
  FromWs : FromWorkspace  Tag=STV FromWs  VariableName=tuvar  SampleTime=0
      SigBuilderData=|
      | common.afterFinalStr = 'Extrapolate'
      | common.sampleTime = 0
      | dataSet(1).timeRange = [0 0.5]
      | dataSet(1).name = 'Group 1'
      | dataSet(2).timeRange = [0 0.5]
      | dataSet(2).name = 'Group 2'
      | dataSet(3).timeRange = [0 1.2]
      | dataSet(3).name = 'Group 3'
      | dataSet(4).timeRange = [0 5]
      | dataSet(4).name = 'Group 4'
      | dataSet(5).timeRange = [0 10]
      | dataSet(5).name = 'Group 5'
      | dataSet(6).timeRange = [0 0.1]
      | dataSet(6).name = 'Group 6'
      | sbobj.Groups(1).Name = 'Group 1'
      | sbobj.Groups(1).Signals.Name = 'call_FordT3McuCfg_Init1'
      | sbobj.Groups(1).Signals.XData = [0 0.001 0.001 0.5]
      | sbobj.Groups(1).Signals.YData = [1 1 0 0]
      | sbobj.Groups(1).TimeRange = [0 0.5]
      | sbobj.Groups(2).Name = 'Group 2'
      | sbobj.Groups(2).Signals.Name = 'call_FordT3McuCfg_Init1'
      | sbobj.Groups(2).Signals.XData = [0 0.001 0.001 0.5]
      | sbobj.Groups(2).Signals.YData = [1 1 0 0]
      | sbobj.Groups(2).TimeRange = [0 0.5]
      | sbobj.Groups(3).Name = 'Group 3'
      | sbobj.Groups(3).Signals.Name = 'call_FordT3McuCfg_Init1'
      | sbobj.Groups(3).Signals.XData = [0 0.001 0.001 1.2]
      | sbobj.Groups(3).Signals.YData = [1 1 0 0]
      | sbobj.Groups(3).TimeRange = [0 1.2]
      | sbobj.Groups(4).Name = 'Group 4'
      | sbobj.Groups(4).Signals.Name = 'call_FordT3McuCfg_Init1'
      | sbobj.Groups(4).Signals.XData = [0 0.001 0.001 5]
      | sbobj.Groups(4).Signals.YData = [1 1 0 0]
      | sbobj.Groups(4).TimeRange = [0 5]
      | sbobj.Groups(5).Name = 'Group 5'
      | sbobj.Groups(5).Signals.Name = 'call_FordT3McuCfg_Init1'
      | sbobj.Groups(5).Signals.XData = [0 0.001 0.001 10]
      | sbobj.Groups(5).Signals.YData = [1 1 0 0]
      | sbobj.Groups(6).Name = 'Group 6'
      | sbobj.Groups(6).Signals.Name = 'call_FordT3McuCfg_Init1'
      | sbobj.Groups(6).Signals.XData = [0 0.001 0.001 0.1]
      | sbobj.Groups(6).Signals.YData = [1 1 0 0]
      | sbobj.Groups(6).TimeRange = [0 0.1]
  call_FordT3McuCfg_Init1 : Outport  Tag=STV Outport
  wires:
  FromWs/1 -> Demux/1
  Demux/1 -> call_FordT3McuCfg_Init1/1

== system CM012A_FordT3McuCfg/Signal Builder1 ==
  Demux : Demux  Tag=STV Demux  Outputs=10
  FromWs : FromWorkspace  Tag=STV FromWs  VariableName=tuvar  SampleTime=0
      SigBuilderData=|
      | common.afterFinalStr = 'Extrapolate'
      | common.sampleTime = 0
      | dataSet.timeRange = [0 2]
      | dataSet.name = 'Group 1'
      | sbobj.Groups.Name = 'Group 1'
      | sbobj.Groups.Signals(1).Name = 'Ia'
      | sbobj.Groups.Signals(1).XData = [0 0.010101010101 0.020202020202 0.030303030303 0.040404040404 0.0505050505051 0.0606060606061 0.0707070707071 0.0808080808081 0.0909090909091 0.10101010101 0.111111111111 ... (199 elements, 1x199)]
      | sbobj.Groups.Signals(1).YData = [1.65 1.75464946743 1.8588775484 1.96226455319 2.06439417885 2.1648551854 2.26324305184 2.35916160495 2.45222461457 2.5420573488 2.62829808294 2.71059955598 ... (199 elements, 1x199)]
      | sbobj.Groups.Signals(2).Name = 'Ib'
      | sbobj.Groups.Signals(2).XData = [0 0.00505050505051 0.010101010101 0.0151515151515 0.020202020202 0.0252525252525 0.030303030303 0.0353535353535 0.040404040404 0.0454545454545 0.0505050505051 0.0555555555556 ... (397 elements, 1x397)]
      | sbobj.Groups.Signals(2).YData = [1.65 1.75464946743 1.8588775484 1.96226455319 2.06439417885 2.1648551854 2.26324305184 2.35916160495 2.45222461457 2.5420573488 2.62829808294 2.71059955598 ... (397 elements, 1x397)]
      | sbobj.Groups.Signals(3).Name = 'Ic'
      | sbobj.Groups.Signals(3).XData = [0 0.0010101010101 0.0020202020202 0.0030303030303 0.0040404040404 0.00505050505051 0.00606060606061 0.00707070707071 0.00808080808081 0.00909090909091 0.010101010101 0.0111111111111 ... (1981 elements, 1x1981)]
      | sbobj.Groups.Signals(3).YData = [1.65 1.75464946743 1.8588775484 1.96226455319 2.06439417885 2.1648551854 2.26324305184 2.35916160495 2.45222461457 2.5420573488 2.62829808294 2.71059955598 ... (1981 elements, 1x1981)]
      | sbobj.Groups.Signals(4).Name = 'Ivtr1Offset'
      | sbobj.Groups.Signals(4).XData = [0 0.010101010101 0.020202020202 0.030303030303 0.040404040404 0.0505050505051 0.0606060606061 0.0707070707071 0.0808080808081 0.0909090909091 0.10101010101 0.111111111111 ... (199 elements, 1x199)]
      | sbobj.Groups.Signals(4).YData = [1.65 1.75464946743 1.8588775484 1.96226455319 2.06439417885 2.1648551854 2.26324305184 2.35916160495 2.45222461457 2.5420573488 2.62829808294 2.71059955598 ... (199 elements, 1x199)]
      | sbobj.Groups.Signals(5).Name = 'ChrgPmpDiag'
      | sbobj.Groups.Signals(5).XData = [0 1 1 2]
      | sbobj.Groups.Signals(5).YData = [0 3.3 0 3.3]
      | sbobj.Groups.Signals(6).Name = 'PwrDiscnctSwtDiag'
      | sbobj.Groups.Signals(6).XData = [0 0.5 0.5 1 1 1.5 1.5 2]
      | sbobj.Groups.Signals(6).YData = [0 3.3 0 3.3 0 3.3 0 3.3]
      | sbobj.Groups.Signals(7).Name = 'EcuT'
      | sbobj.Groups.Signals(7).XData = [0 0.00252525252525 0.00505050505051 0.00757575757576 0.010101010101 0.0126262626263 0.0151515151515 0.0176767676768 0.020202020202 0.0227272727273 0.0252525252525 0.0277777777778 ... (793 elements, 1x793)]
      | sbobj.Groups.Signals(7).YData = [1.65 1.75464946743 1.8588775484 1.96226455319 2.06439417885 2.1648551854 2.26324305184 2.35916160495 2.45222461457 2.5420573488 2.62829808294 2.71059955598 ... (793 elements, 1x793)]
      | sbobj.Groups.Signals(8).Name = 'Vbatt'
      | sbobj.Groups.Signals(8).XData = [0 0.25 0.25 0.5 0.5 0.75 0.75 1 1 1.25 1.25 1.5 1.5 1.75 1.75 2]
      | sbobj.Groups.Signals(8).YData = [0 30 0 30 0 30 0 30 0 30 0 30 0 30 0 30]
      | sbobj.Groups.Signals(9).Name = 'Vswitch'
      | sbobj.Groups.Signals(9).XData = [0 0.0001001001001 0.0002002002002 0.0003003003003 0.0004004004004 0.000500500500501 0.000600600600601 0.000700700700701 0.000800800800801 0.000900900900901 0.001001001001 0.0011011011011 ... (19981 elements, 1x19981)]
      | sbobj.Groups.Signals(9).YData = [8 8.05031546653 8.10062894271 8.15093843828 8.20124196312 8.25153752735 8.30182314143 8.35209681618 8.40235656291 8.45260039347 8.50282632036 8.55303235676 ... (19981 elements, 1x19981)]
      | sbobj.Groups.Signals(10).Name = 'BattRtn'
      | sbobj.Groups.Signals(10).XData = [0 0.025 0.05 0.075 0.1 0.125 0.15 0.175 0.2 0.225 0.25 0.275 0.3 0.325 0.35 0.375 0.4 0.425 0.45 0.475 0.5 0.525 0.55 0.575 0.6 0.625 0.65 0.675 0.7 0.725 0.75 0.775 0.8 0.825 0.85 0.875 0.9 0.925 0.95 0.975 1 1.025 1.05 1.075 1.1 1.125 1.15 1.175 1.2 1.225 1.25 1.275 1.3 1.325 1.35 1.375 1.4 1.425 1.45 1.475 1.5 1.525 1.55 1.575 1.6 1.625 1.65 1.675 1.7 1.725 1.75 1.775 1.8 1.825 1.85 1.875 1.9 1.925 1.95 1.975 2]
      | sbobj.Groups.Signals(10).YData = [1 1.70710678119 2 1.70710678119 1 0.292893218813 0 0.292893218813 1 1.70710678119 2 1.70710678119 1 0.292893218813 0 0.292893218813 1 1.70710678119 2 1.70710678119 1 0.292893218813 0 0.292893218813 1 1.70710678119 2 1.70710678119 1 0.292893218813 0 0.292893218813 1 1.70710678119 2 1.70710678119 1 0.292893218813 0 0.292893218813 1 1.70710678119 2 1.70710678119 1 0.292893218813 0 0.292893218813 1 1.70710678119 2 1.70710678119 1 0.292893218813 0 0.292893218813 1 1.70710678119 2 1.70710678119 1 0.292893218813 0 0.292893218813 1 1.70710678119 2 1.70710678119 1 0.292893218813 0 0.292893218813 1 1.70710678119 2 1.70710678119 1 0.292893218813 0 0.292893218813 1]
      | sbobj.Groups.TimeRange = [0 2]
  Ia : Outport  Tag=STV Outport
  Ib : Outport  Tag=STV Outport  Port=2
  Ic : Outport  Tag=STV Outport  Port=3
  Ivtr1Offset : Outport  Tag=STV Outport  Port=4
  ChrgPmpDiag : Outport  Tag=STV Outport  Port=5
  PwrDiscnctSwtDiag : Outport  Tag=STV Outport  Port=6
  EcuT : Outport  Tag=STV Outport  Port=7
  Vbatt : Outport  Tag=STV Outport  Port=8
  Vswitch : Outport  Tag=STV Outport  Port=9
  BattRtn : Outport  Tag=STV Outport  Port=10
  wires:
  FromWs/1 -> Demux/1
  Demux/1 -> Ia/1
  Demux/2 -> Ib/1
  Demux/3 -> Ic/1
  Demux/4 -> Ivtr1Offset/1
  Demux/5 -> ChrgPmpDiag/1
  Demux/6 -> PwrDiscnctSwtDiag/1
  Demux/7 -> EcuT/1
  Demux/8 -> Vbatt/1
  Demux/9 -> Vswitch/1
  Demux/10 -> BattRtn/1

== system CM012A_FordT3McuCfg/Create Adc0 Raw Results/CopyRight2 ==

== system CM012A_FordT3McuCfg/Create Adc1 Raw Results/CopyRight2 ==

== system CM012A_FordT3McuCfg/FordT3McuCfg/CopyRight2 ==

== system CM012A_FordT3McuCfg/FordT3McuCfg/FordT3McuCfgInit1 ==
  function : TriggerPort  TriggerType=function-call
  CopyRight2 : Subsystem  Description=|  mask(Copyright Information){none=on}
      | Copyright info block.                                               
      |                                                                     
      | Place copyright information at the top of every subsystem in design.
      mask prompts: none "No parameters"
      mask help: Place copyright information at the top of every subsystem in design.
      mask Display:
      | NxtrConf = 'Nexteer Confidential';
      | 
      | sys = bdroot; %handle for the current model ("system")
      | first = get_param(sys,'Created');
      | first = first(end-3:end);  %year is last four digits
      | 
      | last = get_param(sys,'LastModifiedDate');
      | if isempty(last)
      |     last = datestr(now,'yyyy');
      | else
      |     last = last(end-3:end);
      | end
      | 
      | if strcmp(first,last)
      |     fprintf('%s -- Copyright %s Nexteer',NxtrConf,first)
      | else
      |     fprintf('%s -- %s%s- %s Nexteer',NxtrConf,char(169),first,last)
      | end
  Register Initialization : Subsystem  Priority=10
      settings: AttributesFormatString=Priority: %<Priority>

== system CM012A_FordT3McuCfg/FordT3McuCfg/FordT3McuCfgInit2 ==
  function : TriggerPort  TriggerType=function-call
  CopyRight2 : Subsystem  Description=|  mask(Copyright Information){none=on}
      | Copyright info block.                                               
      |                                                                     
      | Place copyright information at the top of every subsystem in design.
      mask prompts: none "No parameters"
      mask help: Place copyright information at the top of every subsystem in design.
      mask Display:
      | NxtrConf = 'Nexteer Confidential';
      | 
      | sys = bdroot; %handle for the current model ("system")
      | first = get_param(sys,'Created');
      | first = first(end-3:end);  %year is last four digits
      | 
      | last = get_param(sys,'LastModifiedDate');
      | if isempty(last)
      |     last = datestr(now,'yyyy');
      | else
      |     last = last(end-3:end);
      | end
      | 
      | if strcmp(first,last)
      |     fprintf('%s -- Copyright %s Nexteer',NxtrConf,first)
      | else
      |     fprintf('%s -- %s%s- %s Nexteer',NxtrConf,char(169),first,last)
      | end
  Register Initialization : Subsystem  Priority=10
      settings: AttributesFormatString=Priority: %<Priority>

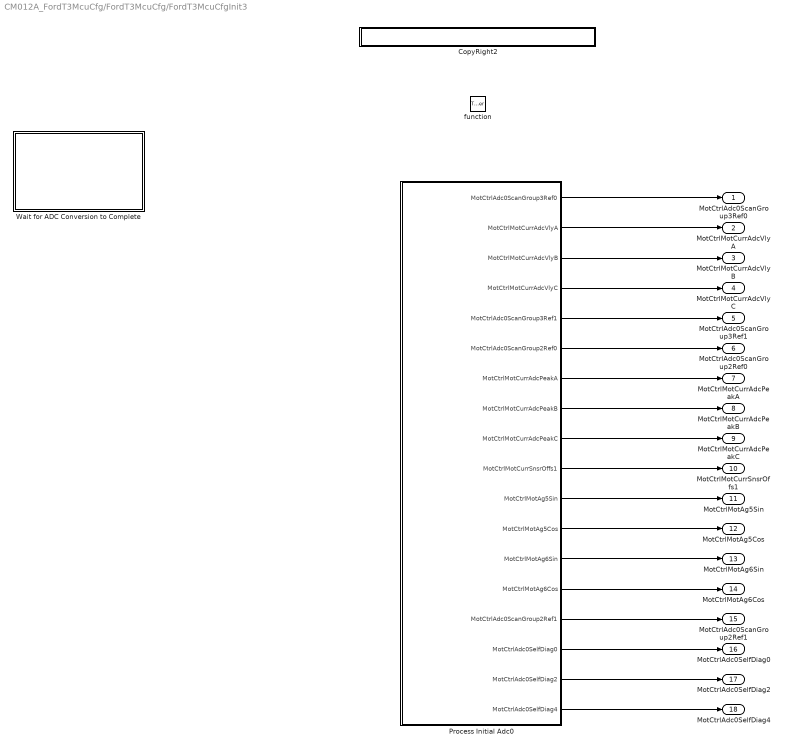
== system CM012A_FordT3McuCfg/FordT3McuCfg/FordT3McuCfgInit3 ==
  function : TriggerPort  TriggerType=function-call
  CopyRight2 : Subsystem  Description=|  mask(Copyright Information){none=on}
      | Copyright info block.                                               
      |                                                                     
      | Place copyright information at the top of every subsystem in design.
      mask prompts: none "No parameters"
      mask help: Place copyright information at the top of every subsystem in design.
      mask Display:
      | NxtrConf = 'Nexteer Confidential';
      | 
      | sys = bdroot; %handle for the current model ("system")
      | first = get_param(sys,'Created');
      | first = first(end-3:end);  %year is last four digits
      | 
      | last = get_param(sys,'LastModifiedDate');
      | if isempty(last)
      |     last = datestr(now,'yyyy');
      | else
      |     last = last(end-3:end);
      | end
      | 
      | if strcmp(first,last)
      |     fprintf('%s -- Copyright %s Nexteer',NxtrConf,first)
      | else
      |     fprintf('%s -- %s%s- %s Nexteer',NxtrConf,char(169),first,last)
      | end
  Process Initial Adc0 : Subsystem  RequirementInfo={} %GIDa_d862d82c_969a_40be_9cba_5dad28e4f649  Priority=20
      settings: AttributesFormatString=Priority: %<Priority>
  Wait for ADC Conversion to Complete : Subsystem  Priority=10
      settings: AttributesFormatString=Priority: %<Priority>
  MotCtrlAdc0ScanGroup3Ref0 : Outport
  MotCtrlMotCurrAdcVlyA : Outport  Port=2
  MotCtrlMotCurrAdcVlyB : Outport  Port=3
  MotCtrlMotCurrAdcVlyC : Outport  Port=4
  MotCtrlAdc0ScanGroup3Ref1 : Outport  Port=5
  MotCtrlAdc0ScanGroup2Ref0 : Outport  Port=6
  MotCtrlMotCurrAdcPeakA : Outport  Port=7
  MotCtrlMotCurrAdcPeakB : Outport  Port=8
  MotCtrlMotCurrAdcPeakC : Outport  Port=9
  MotCtrlMotCurrSnsrOffs1 : Outport  Port=10
  MotCtrlMotAg5Sin : Outport  Port=11
  MotCtrlMotAg5Cos : Outport  Port=12
  MotCtrlMotAg6Sin : Outport  Port=13
  MotCtrlMotAg6Cos : Outport  Port=14
  MotCtrlAdc0ScanGroup2Ref1 : Outport  Port=15
  MotCtrlAdc0SelfDiag0 : Outport  Port=16
  MotCtrlAdc0SelfDiag2 : Outport  Port=17
  MotCtrlAdc0SelfDiag4 : Outport  Port=18
  wires:
  Process Initial Adc0/1(MotCtrlAdc0ScanGroup3Ref0) -> MotCtrlAdc0ScanGroup3Ref0/1
  Process Initial Adc0/2(MotCtrlMotCurrAdcVlyA) -> MotCtrlMotCurrAdcVlyA/1
  Process Initial Adc0/3(MotCtrlMotCurrAdcVlyB) -> MotCtrlMotCurrAdcVlyB/1
  Process Initial Adc0/4(MotCtrlMotCurrAdcVlyC) -> MotCtrlMotCurrAdcVlyC/1
  Process Initial Adc0/5(MotCtrlAdc0ScanGroup3Ref1) -> MotCtrlAdc0ScanGroup3Ref1/1
  Process Initial Adc0/6(MotCtrlAdc0ScanGroup2Ref0) -> MotCtrlAdc0ScanGroup2Ref0/1
  Process Initial Adc0/7(MotCtrlMotCurrAdcPeakA) -> MotCtrlMotCurrAdcPeakA/1
  Process Initial Adc0/8(MotCtrlMotCurrAdcPeakB) -> MotCtrlMotCurrAdcPeakB/1
  Process Initial Adc0/9(MotCtrlMotCurrAdcPeakC) -> MotCtrlMotCurrAdcPeakC/1
  Process Initial Adc0/10(MotCtrlMotCurrSnsrOffs1) -> MotCtrlMotCurrSnsrOffs1/1
  Process Initial Adc0/11(MotCtrlMotAg5Sin) -> MotCtrlMotAg5Sin/1
  Process Initial Adc0/14(MotCtrlMotAg6Cos) -> MotCtrlMotAg6Cos/1
  Process Initial Adc0/13(MotCtrlMotAg6Sin) -> MotCtrlMotAg6Sin/1
  Process Initial Adc0/12(MotCtrlMotAg5Cos) -> MotCtrlMotAg5Cos/1
  Process Initial Adc0/15(MotCtrlAdc0ScanGroup2Ref1) -> MotCtrlAdc0ScanGroup2Ref1/1
  Process Initial Adc0/16(MotCtrlAdc0SelfDiag0) -> MotCtrlAdc0SelfDiag0/1
  Process Initial Adc0/18(MotCtrlAdc0SelfDiag4) -> MotCtrlAdc0SelfDiag4/1
  Process Initial Adc0/17(MotCtrlAdc0SelfDiag2) -> MotCtrlAdc0SelfDiag2/1

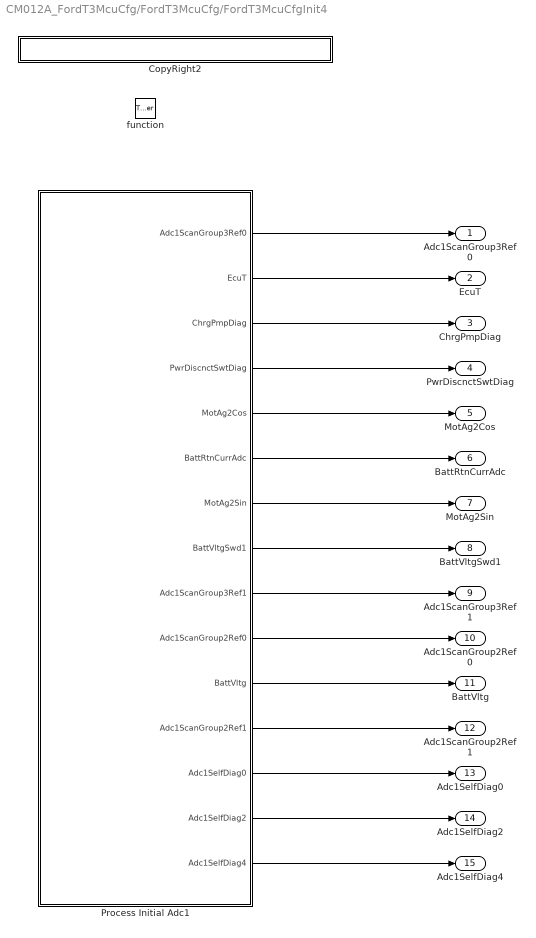
== system CM012A_FordT3McuCfg/FordT3McuCfg/FordT3McuCfgInit4 ==
  function : TriggerPort  TriggerType=function-call
  CopyRight2 : Subsystem  Description=|  mask(Copyright Information){none=on}
      | Copyright info block.                                               
      |                                                                     
      | Place copyright information at the top of every subsystem in design.
      mask prompts: none "No parameters"
      mask help: Place copyright information at the top of every subsystem in design.
      mask Display:
      | NxtrConf = 'Nexteer Confidential';
      | 
      | sys = bdroot; %handle for the current model ("system")
      | first = get_param(sys,'Created');
      | first = first(end-3:end);  %year is last four digits
      | 
      | last = get_param(sys,'LastModifiedDate');
      | if isempty(last)
      |     last = datestr(now,'yyyy');
      | else
      |     last = last(end-3:end);
      | end
      | 
      | if strcmp(first,last)
      |     fprintf('%s -- Copyright %s Nexteer',NxtrConf,first)
      | else
      |     fprintf('%s -- %s%s- %s Nexteer',NxtrConf,char(169),first,last)
      | end
  Process Initial Adc1 : Subsystem  RequirementInfo={} %GIDa_376048c3_94d2_40f9_9974_227dea3c5b4f  Priority=40
      settings: AttributesFormatString=Priority: %<Priority>
  Adc1ScanGroup3Ref0 : Outport
  EcuT : Outport  Port=2
  ChrgPmpDiag : Outport  Port=3
  PwrDiscnctSwtDiag : Outport  Port=4
  MotAg2Cos : Outport  Port=5
  BattRtnCurrAdc : Outport  Port=6
  MotAg2Sin : Outport  Port=7
  BattVltgSwd1 : Outport  Port=8
  Adc1ScanGroup3Ref1 : Outport  Port=9
  Adc1ScanGroup2Ref0 : Outport  Port=10
  BattVltg : Outport  Port=11
  Adc1ScanGroup2Ref1 : Outport  Port=12
  Adc1SelfDiag0 : Outport  Port=13
  Adc1SelfDiag2 : Outport  Port=14
  Adc1SelfDiag4 : Outport  Port=15
  wires:
  Process Initial Adc1/1(Adc1ScanGroup3Ref0) -> Adc1ScanGroup3Ref0/1
  Process Initial Adc1/2(EcuT) -> EcuT/1
  Process Initial Adc1/3(ChrgPmpDiag) -> ChrgPmpDiag/1
  Process Initial Adc1/4(PwrDiscnctSwtDiag) -> PwrDiscnctSwtDiag/1
  Process Initial Adc1/5(MotAg2Cos) -> MotAg2Cos/1
  Process Initial Adc1/6(BattRtnCurrAdc) -> BattRtnCurrAdc/1
  Process Initial Adc1/7(MotAg2Sin) -> MotAg2Sin/1
  Process Initial Adc1/8(BattVltgSwd1) -> BattVltgSwd1/1
  Process Initial Adc1/9(Adc1ScanGroup3Ref1) -> Adc1ScanGroup3Ref1/1
  Process Initial Adc1/10(Adc1ScanGroup2Ref0) -> Adc1ScanGroup2Ref0/1
  Process Initial Adc1/11(BattVltg) -> BattVltg/1
  Process Initial Adc1/14(Adc1SelfDiag2) -> Adc1SelfDiag2/1
  Process Initial Adc1/15(Adc1SelfDiag4) -> Adc1SelfDiag4/1
  Process Initial Adc1/13(Adc1SelfDiag0) -> Adc1SelfDiag0/1
  Process Initial Adc1/12(Adc1ScanGroup2Ref1) -> Adc1ScanGroup2Ref1/1

== system CM012A_FordT3McuCfg/FordT3McuCfg/FordT3McuCfgInit5 ==
  EcuId : Inport
  function : TriggerPort  TriggerType=function-call
  CopyRight2 : Subsystem  Description=|  mask(Copyright Information){none=on}
      | Copyright info block.                                               
      |                                                                     
      | Place copyright information at the top of every subsystem in design.
      mask prompts: none "No parameters"
      mask help: Place copyright information at the top of every subsystem in design.
      mask Display:
      | NxtrConf = 'Nexteer Confidential';
      | 
      | sys = bdroot; %handle for the current model ("system")
      | first = get_param(sys,'Created');
      | first = first(end-3:end);  %year is last four digits
      | 
      | last = get_param(sys,'LastModifiedDate');
      | if isempty(last)
      |     last = datestr(now,'yyyy');
      | else
      |     last = last(end-3:end);
      | end
      | 
      | if strcmp(first,last)
      |     fprintf('%s -- Copyright %s Nexteer',NxtrConf,first)
      | else
      |     fprintf('%s -- %s%s- %s Nexteer',NxtrConf,char(169),first,last)
      | end
  If : If  IfExpression=u1 == 1
      settings: AttributesFormatString=|
      | %<IfExpression>
      | %<ElseIfExpressions>
  If Action Subsystem : Subsystem  TreatAsAtomicUnit=on
  If Action Subsystem3 : Subsystem  TreatAsAtomicUnit=on
  Merge : Merge
  Merge1 : Merge
  Merge2 : Merge
  HwAg1SnsrTyp : Outport
  HwAg1SnsrNr : Outport  Port=2  OutDataTypeStr=uint8
  MotAg2MeasOffs : Outport  Port=3
  wires:
  EcuId/1 -> If/1
  If/1 -> If Action Subsystem/Action
  If/2 -> If Action Subsystem3/Action
  If Action Subsystem/1(HwAg1SnsrTyp) -> Merge/1
  If Action Subsystem3/1(HwAg1SnsrTyp) -> Merge/2
  If Action Subsystem/2(HwAg1SnsrNr) -> Merge1/1
  If Action Subsystem3/2(HwAg1SnsrNr) -> Merge1/2
  Merge/1 -> HwAg1SnsrTyp/1
  Merge1/1 -> HwAg1SnsrNr/1
  If Action Subsystem/3(MotAg2MeasOffs) -> Merge2/1
  If Action Subsystem3/3(MotAg2MeasOffs) -> Merge2/2
  Merge2/1 -> MotAg2MeasOffs/1

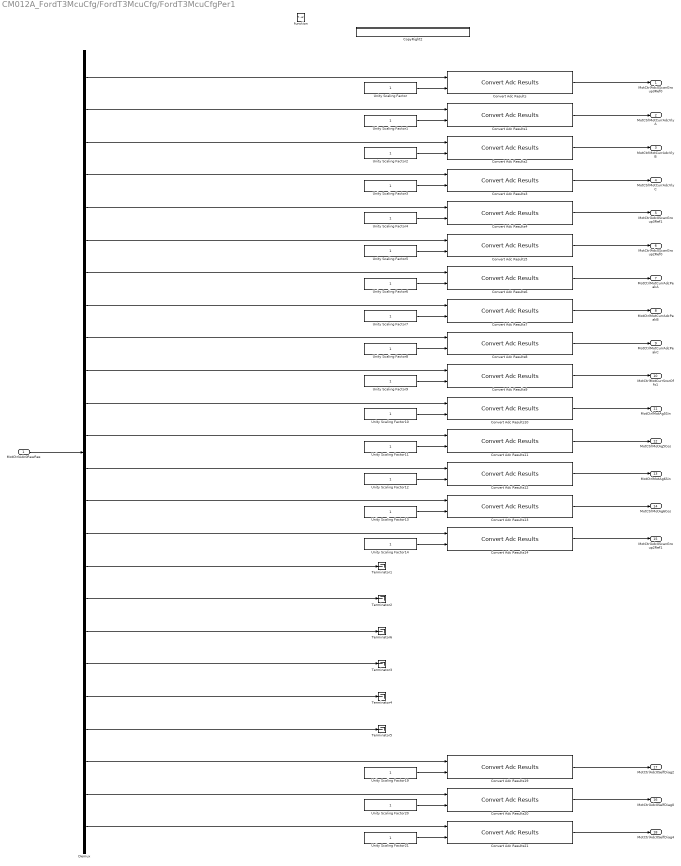
== system CM012A_FordT3McuCfg/FordT3McuCfg/FordT3McuCfgPer1 ==
  MotCtrlAdc0RawRes : Inport
  function : TriggerPort  TriggerType=function-call
  Convert Adc Results{,4..5,14,19..21} (7 alike) : CM012A_FordT3McuCfg_ModelLibrary/Convert Adc Results
  Convert Adc Results1 : CM012A_FordT3McuCfg_ModelLibrary/Convert Adc Results  RequirementInfo="{'linktype_rmi_doors' '00016ba8 (/ESG Group/FDD Module Requirements/EA4 Specific/CM012A_FordT3McuCfg)' '#CM012A_38' 'true' 'REQ:  CM012A_38' '' } %GIDa_d68b8fc1_7709_4618_b80e_8796169f479b"
  Convert Adc Results10 : CM012A_FordT3McuCfg_ModelLibrary/Convert Adc Results  RequirementInfo="{'linktype_rmi_doors' '00016ba8 (/ESG Group/FDD Module Requirements/EA4 Specific/CM012A_FordT3McuCfg)' '#CM012A_174' 'true' 'REQ:  CM012A_174' '' } %GIDa_78acc9b1_0c35_4fa0_9187_4ce9060727c9"
  Convert Adc Results11 : CM012A_FordT3McuCfg_ModelLibrary/Convert Adc Results  RequirementInfo="{'linktype_rmi_doors' '00016ba8 (/ESG Group/FDD Module Requirements/EA4 Specific/CM012A_FordT3McuCfg)' '#CM012A_175' 'true' 'REQ:  CM012A_175' '' } %GIDa_72ea0b38_0716_4b32_a7fa_0bfeaedc5d3b"
  Convert Adc Results12 : CM012A_FordT3McuCfg_ModelLibrary/Convert Adc Results  RequirementInfo="{'linktype_rmi_doors' '00016ba8 (/ESG Group/FDD Module Requirements/EA4 Specific/CM012A_FordT3McuCfg)' '#CM012A_176' 'true' 'REQ:  CM012A_176' '' } %GIDa_db215c6c_10f6_460c_b71f_201c0c4481fc"
  Convert Adc Results13 : CM012A_FordT3McuCfg_ModelLibrary/Convert Adc Results  RequirementInfo="{'linktype_rmi_doors' '00016ba8 (/ESG Group/FDD Module Requirements/EA4 Specific/CM012A_FordT3McuCfg)' '#CM012A_177' 'true' 'REQ:  CM012A_177' '' } %GIDa_18503211_4668_4601_9683_14c602fa2bc8"
  Convert Adc Results2 : CM012A_FordT3McuCfg_ModelLibrary/Convert Adc Results  RequirementInfo="{'linktype_rmi_doors' '00016ba8 (/ESG Group/FDD Module Requirements/EA4 Specific/CM012A_FordT3McuCfg)' '#CM012A_122' 'true' 'REQ:  CM012A_122' '' } %GIDa_0fee4947_1a8b_4e3c_ace4_e216b5f36d5c"
  Convert Adc Results3 : CM012A_FordT3McuCfg_ModelLibrary/Convert Adc Results  RequirementInfo="{'linktype_rmi_doors' '00016ba8 (/ESG Group/FDD Module Requirements/EA4 Specific/CM012A_FordT3McuCfg)' '#CM012A_126' 'true' 'REQ:  CM012A_126' '' } %GIDa_e29479a4_0cf4_445a_8199_5ef2b1401b8f"
  Convert Adc Results6 : CM012A_FordT3McuCfg_ModelLibrary/Convert Adc Results  RequirementInfo="{'linktype_rmi_doors' '00016ba8 (/ESG Group/FDD Module Requirements/EA4 Specific/CM012A_FordT3McuCfg)' '#CM012A_170' 'true' 'REQ:  CM012A_170' '' } %GIDa_d2a642ed_f8de_4b26_b4aa_32a988825931"
  Convert Adc Results7 : CM012A_FordT3McuCfg_ModelLibrary/Convert Adc Results  RequirementInfo="{'linktype_rmi_doors' '00016ba8 (/ESG Group/FDD Module Requirements/EA4 Specific/CM012A_FordT3McuCfg)' '#CM012A_171' 'true' 'REQ:  CM012A_171' '' } %GIDa_e8368225_2f11_4b2c_9ab6_44d6352a484e"
  Convert Adc Results8 : CM012A_FordT3McuCfg_ModelLibrary/Convert Adc Results  RequirementInfo="{'linktype_rmi_doors' '00016ba8 (/ESG Group/FDD Module Requirements/EA4 Specific/CM012A_FordT3McuCfg)' '#CM012A_172' 'true' 'REQ:  CM012A_172' '' } %GIDa_5bfdc6dc_be49_45fd_aae1_e3fe4f14c744"
  Convert Adc Results9 : CM012A_FordT3McuCfg_ModelLibrary/Convert Adc Results  RequirementInfo="{'linktype_rmi_doors' '00016ba8 (/ESG Group/FDD Module Requirements/EA4 Specific/CM012A_FordT3McuCfg)' '#CM012A_173' 'true' 'REQ:  CM012A_173' '' } %GIDa_d3aff69a_1839_4954_b3ad_b41858deb123"
  CopyRight2 : Subsystem  Description=|  mask(Copyright Information){none=on}
      | Copyright info block.                                               
      |                                                                     
      | Place copyright information at the top of every subsystem in design.
      mask prompts: none "No parameters"
      mask help: Place copyright information at the top of every subsystem in design.
      mask Display:
      | NxtrConf = 'Nexteer Confidential';
      | 
      | sys = bdroot; %handle for the current model ("system")
      | first = get_param(sys,'Created');
      | first = first(end-3:end);  %year is last four digits
      | 
      | last = get_param(sys,'LastModifiedDate');
      | if isempty(last)
      |     last = datestr(now,'yyyy');
      | else
      |     last = last(end-3:end);
      | end
      | 
      | if strcmp(first,last)
      |     fprintf('%s -- Copyright %s Nexteer',NxtrConf,first)
      | else
      |     fprintf('%s -- %s%s- %s Nexteer',NxtrConf,char(169),first,last)
      | end
  Demux : Demux  Outputs=24
  Terminator{1..6} (6 alike) : Terminator
  Unity Scaling Factor{,1..14,19..21} (18 alike) : Constant  OutDataTypeStr=single
  MotCtrlAdc0ScanGroup3Ref0 : Outport
  MotCtrlMotCurrAdcVlyA : Outport  Port=2
  MotCtrlMotCurrAdcVlyB : Outport  Port=3
  MotCtrlMotCurrAdcVlyC : Outport  Port=4
  MotCtrlAdc0ScanGroup3Ref1 : Outport  Port=5
  MotCtrlAdc0ScanGroup2Ref0 : Outport  Port=6
  MotCtrlMotCurrAdcPeakA : Outport  Port=7
  MotCtrlMotCurrAdcPeakB : Outport  Port=8
  MotCtrlMotCurrAdcPeakC : Outport  Port=9
  MotCtrlMotCurrSnsrOffs1 : Outport  Port=10
  MotCtrlMotAg5Sin : Outport  Port=11
  MotCtrlMotAg5Cos : Outport  Port=12
  MotCtrlMotAg6Sin : Outport  Port=13
  MotCtrlMotAg6Cos : Outport  Port=14
  MotCtrlAdc0ScanGroup2Ref1 : Outport  Port=15
  MotCtrlAdc0SelfDiag0 : Outport  Port=16
  MotCtrlAdc0SelfDiag2 : Outport  Port=17
  MotCtrlAdc0SelfDiag4 : Outport  Port=18
  wires:
  MotCtrlAdc0RawRes/1 -> Demux/1
  Unity Scaling Factor/1 -> Convert Adc Results/2
  Unity Scaling Factor1/1 -> Convert Adc Results1/2
  Unity Scaling Factor2/1 -> Convert Adc Results2/2
  Unity Scaling Factor3/1 -> Convert Adc Results3/2
  Unity Scaling Factor4/1 -> Convert Adc Results4/2
  Unity Scaling Factor5/1 -> Convert Adc Results5/2
  Unity Scaling Factor6/1 -> Convert Adc Results6/2
  Unity Scaling Factor7/1 -> Convert Adc Results7/2
  Unity Scaling Factor8/1 -> Convert Adc Results8/2
  Unity Scaling Factor19/1 -> Convert Adc Results19/2
  Unity Scaling Factor20/1 -> Convert Adc Results20/2
  Unity Scaling Factor21/1 -> Convert Adc Results21/2
  Demux/4 -> Convert Adc Results3/1
  Demux/24 -> Convert Adc Results21/1
  Demux/23 -> Convert Adc Results20/1
  Demux/22 -> Convert Adc Results19/1
  Demux/21 -> Terminator5/1
  Demux/19 -> Terminator3/1
  Demux/20 -> Terminator4/1
  Demux/9 -> Convert Adc Results8/1
  Demux/7 -> Convert Adc Results6/1
  Demux/8 -> Convert Adc Results7/1
  Demux/5 -> Convert Adc Results4/1
  Demux/6 -> Convert Adc Results5/1
  Unity Scaling Factor9/1 -> Convert Adc Results9/2
  Unity Scaling Factor10/1 -> Convert Adc Results10/2
  Unity Scaling Factor11/1 -> Convert Adc Results11/2
  Unity Scaling Factor12/1 -> Convert Adc Results12/2
  Unity Scaling Factor13/1 -> Convert Adc Results13/2
  Unity Scaling Factor14/1 -> Convert Adc Results14/2
  Demux/10 -> Convert Adc Results9/1
  Demux/15 -> Convert Adc Results14/1
  Demux/13 -> Convert Adc Results12/1
  Demux/14 -> Convert Adc Results13/1
  Demux/11 -> Convert Adc Results10/1
  Demux/12 -> Convert Adc Results11/1
  Demux/1 -> Convert Adc Results/1
  Demux/2 -> Convert Adc Results1/1
  Demux/3 -> Convert Adc Results2/1
  Convert Adc Results2/1 -> MotCtrlMotCurrAdcVlyB/1
  Convert Adc Results3/1 -> MotCtrlMotCurrAdcVlyC/1
  Convert Adc Results4/1 -> MotCtrlAdc0ScanGroup3Ref1/1
  Convert Adc Results5/1 -> MotCtrlAdc0ScanGroup2Ref0/1
  Convert Adc Results6/1 -> MotCtrlMotCurrAdcPeakA/1
  Convert Adc Results7/1 -> MotCtrlMotCurrAdcPeakB/1
  Convert Adc Results8/1 -> MotCtrlMotCurrAdcPeakC/1
  Convert Adc Results9/1 -> MotCtrlMotCurrSnsrOffs1/1
  Convert Adc Results10/1 -> MotCtrlMotAg5Sin/1
  Convert Adc Results13/1 -> MotCtrlMotAg6Cos/1
  Convert Adc Results12/1 -> MotCtrlMotAg6Sin/1
  Convert Adc Results11/1 -> MotCtrlMotAg5Cos/1
  Convert Adc Results14/1 -> MotCtrlAdc0ScanGroup2Ref1/1
  Convert Adc Results/1 -> MotCtrlAdc0ScanGroup3Ref0/1
  Convert Adc Results1/1 -> MotCtrlMotCurrAdcVlyA/1
  Demux/18 -> Terminator6/1
  Demux/16 -> Terminator1/1
  Demux/17 -> Terminator2/1
  Convert Adc Results20/1 -> MotCtrlAdc0SelfDiag0/1
  Convert Adc Results19/1 -> MotCtrlAdc0SelfDiag2/1
  Convert Adc Results21/1 -> MotCtrlAdc0SelfDiag4/1
